simulink library "threephase_voltage_current_measure"  (R2025b)
settings: Solver=VariableStepAuto  StartTime=0.0  StopTime=10.0  RelTol=1e-3
libraries: fl_lib x12, nesl_utility x9
settings Model: Creator=ltnbda  LastModifiedBy=ltnbda

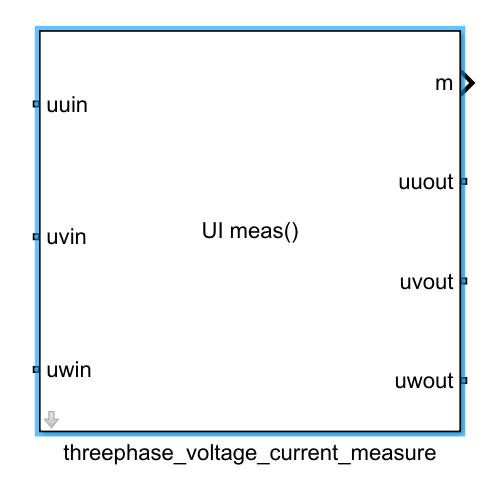
[thumbnail: Simulink's stored preview of the top-level diagram]
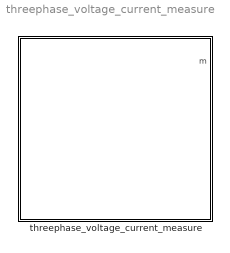
== system threephase_voltage_current_measure ==
  threephase_voltage_current_measure : Subsystem
      mask Display:
      | disp('UI meas()');
      | 
      | port_label('lconn', 1, 'uuin');
      | port_label('lconn', 2, 'uvin');
      | port_label('lconn', 3, 'uwin');
      | 
      | port_label('rconn', 1, 'uuout');
      | port_label('rconn', 2, 'uvout');
      | port_label('rconn', 3, 'uwout');
      | 
      | port_label('output', 1, 'm');

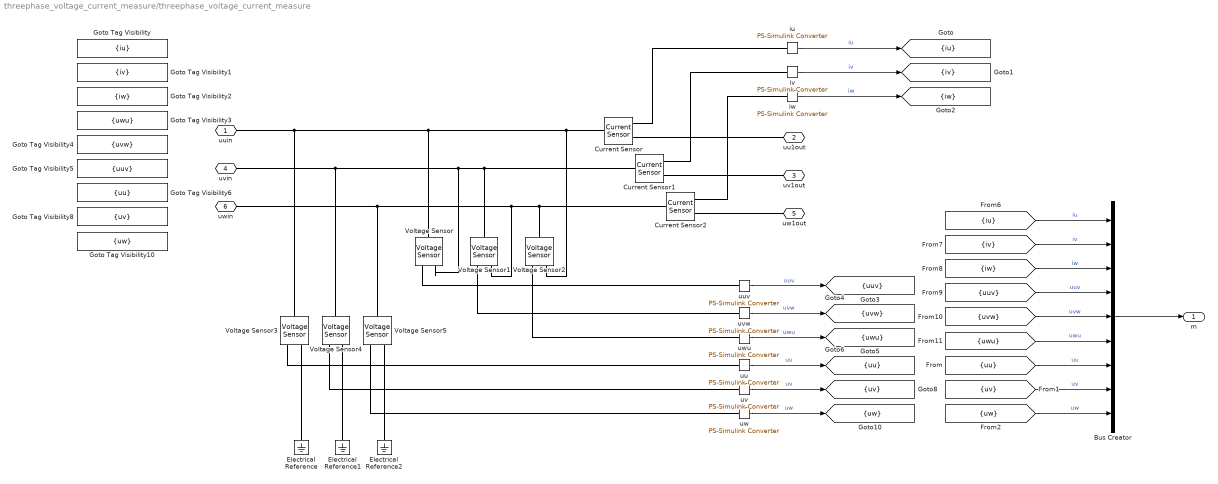
== system threephase_voltage_current_measure/threephase_voltage_current_measure ==
  Bus Creator : BusCreator  Inputs=9
  Current Sensor : fl_lib/Electrical/Electrical Sensors/Current Sensor
  Current Sensor1 : fl_lib/Electrical/Electrical Sensors/Current Sensor
  Current Sensor2 : fl_lib/Electrical/Electrical Sensors/Current Sensor
  Electrical Reference : fl_lib/Electrical/Electrical Elements/Electrical Reference
  Electrical Reference1 : fl_lib/Electrical/Electrical Elements/Electrical Reference
  Electrical Reference2 : fl_lib/Electrical/Electrical Elements/Electrical Reference
  Goto Tag Visibility : GotoTagVisibility  GotoTag=iu
  Goto Tag Visibility1 : GotoTagVisibility  GotoTag=iv
  Goto Tag Visibility10 : GotoTagVisibility  GotoTag=uw
  Goto Tag Visibility2 : GotoTagVisibility  GotoTag=iw
  Goto Tag Visibility3 : GotoTagVisibility  GotoTag=uwu
  Goto Tag Visibility4 : GotoTagVisibility  GotoTag=uvw
  Goto Tag Visibility5 : GotoTagVisibility  GotoTag=uuv
  Goto Tag Visibility6 : GotoTagVisibility  GotoTag=uu
  Goto Tag Visibility8 : GotoTagVisibility  GotoTag=uv
  Voltage Sensor{,1..5} (6 alike) : fl_lib/Electrical/Electrical Sensors/Voltage Sensor
  iu : nesl_utility/PS-Simulink Converter  PhysicalDomain=network_engine_domain  SubClassName=ps_output  LeftPortType=input  RightPortType=output  PseudoPeriodic=off  Frequencies=[]  VectorFormat=1-D array  Unit=A  AffineConversion=off
  iv : nesl_utility/PS-Simulink Converter  PhysicalDomain=network_engine_domain  SubClassName=ps_output  LeftPortType=input  RightPortType=output  PseudoPeriodic=off  Frequencies=[]  VectorFormat=1-D array  Unit=A  AffineConversion=off
  iw : nesl_utility/PS-Simulink Converter  PhysicalDomain=network_engine_domain  SubClassName=ps_output  LeftPortType=input  RightPortType=output  PseudoPeriodic=off  Frequencies=[]  VectorFormat=1-D array  Unit=A  AffineConversion=off
  uu : nesl_utility/PS-Simulink Converter  PhysicalDomain=network_engine_domain  SubClassName=ps_output  LeftPortType=input  RightPortType=output  PseudoPeriodic=off  Frequencies=[]  VectorFormat=1-D array  Unit=V  AffineConversion=off
  uuv : nesl_utility/PS-Simulink Converter  PhysicalDomain=network_engine_domain  SubClassName=ps_output  LeftPortType=input  RightPortType=output  PseudoPeriodic=off  Frequencies=[]  VectorFormat=1-D array  Unit=V  AffineConversion=off
  uv : nesl_utility/PS-Simulink Converter  PhysicalDomain=network_engine_domain  SubClassName=ps_output  LeftPortType=input  RightPortType=output  PseudoPeriodic=off  Frequencies=[]  VectorFormat=1-D array  Unit=V  AffineConversion=off
  uvw : nesl_utility/PS-Simulink Converter  PhysicalDomain=network_engine_domain  SubClassName=ps_output  LeftPortType=input  RightPortType=output  PseudoPeriodic=off  Frequencies=[]  VectorFormat=1-D array  Unit=V  AffineConversion=off
  uw : nesl_utility/PS-Simulink Converter  PhysicalDomain=network_engine_domain  SubClassName=ps_output  LeftPortType=input  RightPortType=output  PseudoPeriodic=off  Frequencies=[]  VectorFormat=1-D array  Unit=V  AffineConversion=off
  uwu : nesl_utility/PS-Simulink Converter  PhysicalDomain=network_engine_domain  SubClassName=ps_output  LeftPortType=input  RightPortType=output  PseudoPeriodic=off  Frequencies=[]  VectorFormat=1-D array  Unit=V  AffineConversion=off
  uuin : PMIOPort  Side=Left
  uu1out : PMIOPort  Port=2  Side=Right
  uv1out : PMIOPort  Port=3  Side=Right
  uvin : PMIOPort  Port=4  Side=Left
  uw1out : PMIOPort  Port=5  Side=Right
  uwin : PMIOPort  Port=6  Side=Left
  m : Outport
  tag scope: iu=scoped, iv=scoped, iw=scoped, uu=scoped, uuv=scoped, uv=scoped, uvw=scoped, uw=scoped, uwu=scoped
  wires:
  iu/1 -> [iu]  "iu"
  iv/1 -> [iv]  "iv"
  iw/1 -> [iw]  "iw"
  uvw/1 -> [uvw]  "uvw"
  uuv/1 -> [uuv]  "uuv"
  uwu/1 -> [uwu]  "uwu"
  uu/1 -> [uu]  "uu"
  uv/1 -> [uv]  "uv"
  uw/1 -> [uw]  "uw"
  Bus Creator/1 -> m/1
  [iu] -> Bus Creator/1  "iu"
  [uw] -> Bus Creator/9  "uw"
  [uv] -> Bus Creator/8  "uv"
  [uu] -> Bus Creator/7  "uu"
  [uwu] -> Bus Creator/6  "uwu"
  [uvw] -> Bus Creator/5  "uvw"
  [uuv] -> Bus Creator/4  "uuv"
  [iw] -> Bus Creator/3  "iw"
  [iv] -> Bus Creator/2  "iv"
  connections:
  Voltage Sensor1/LConn1 -- Current Sensor1/LConn1 -- uvin/RConn1 -- Voltage Sensor4/LConn1 -- Voltage Sensor/RConn2
  Voltage Sensor/RConn1 -- uuv/LConn1
  Current Sensor/RConn2 -- uu1out/RConn1
  Voltage Sensor1/RConn1 -- uvw/LConn1
  Current Sensor2/LConn1 -- Voltage Sensor1/RConn2 -- uwin/RConn1 -- Voltage Sensor5/LConn1 -- Voltage Sensor2/LConn1
  Voltage Sensor/LConn1 -- Voltage Sensor2/RConn2 -- Current Sensor/LConn1 -- Voltage Sensor3/LConn1 -- uuin/RConn1
  Current Sensor1/RConn2 -- uv1out/RConn1
  Voltage Sensor2/RConn1 -- uwu/LConn1
  iv/LConn1 -- Current Sensor1/RConn1
  iu/LConn1 -- Current Sensor/RConn1
  iw/LConn1 -- Current Sensor2/RConn1
  Current Sensor2/RConn2 -- uw1out/RConn1
  Voltage Sensor3/RConn2 -- Electrical Reference/LConn1
  Voltage Sensor4/RConn2 -- Electrical Reference1/LConn1
  Voltage Sensor5/RConn2 -- Electrical Reference2/LConn1
  uv/LConn1 -- Voltage Sensor4/RConn1
  uw/LConn1 -- Voltage Sensor5/RConn1
  Voltage Sensor3/RConn1 -- uu/LConn1
